simulink model "tp414070"  (Simulink 3.0)
settings: Solver=ode1  SolverMode=SingleTasking  StartTime=0.0  StopTime=t_sim  FixedStep=Ts  RelTol=1e-3
values from neighbouring files (symbols this model uses):
  d_action_on = 1    [init_PID1_windupless_tune3.m]
  i_action_on = 1    [init_PID1_windupless_tune3.m]
  Ks = input('Put integrator gain value Ks = ')    [init_PI1_windupless.m]    (also in init_PID1_windupless_tune3.m)
  P = input('Put gain of P component = ')    [init_PI1_windupless.m]    (also in init_PID1_windupless_tune3.m; init_step_resp2.m = 2)
  T1 = input('Put time constant T1 value = ')    [init_PID1_windupless_tune3.m]
  Tfd = input('feasibility and filtration (T1/5) = ')    [init_PID1_windupless_tune3.m]
  Tfil = input('Put time constant Tfil of inner loop = ')    [init_PI1_windupless.m]    (also in init_PID1_windupless_tune3.m)
  Ts = 1    [init_PI1_windupless.m]    (also in init_PID1_windupless_tune3.m = 0.5; init_step_resp2.m = 0.2; prev45_0.mat = 0.2; prev45_1.mat = 0.2)
  Umax = 5    [init_PI1_windupless.m]    (also in init_PID1_windupless_tune3.m; init_step_resp2.m; prev45_0.mat; prev45_1.mat)
  Umin = 0    [init_PI1_windupless.m]    (also in init_PID1_windupless_tune3.m; init_step_resp2.m; prev45_0.mat; prev45_1.mat)
libraries: udaq28LT_lib x1
settings Model: LastModifiedBy=mato  ExtModeMexFile=rtwinext  ExtModeTrigDuration=100000  SaveFormat=Matrix  RTWSystemTargetFile=rtwin.tlc  RTWTemplateMakefile=rtwintmf  RTWOptions="-aCCOptimize=1 -aEnforceIntegerDowncast=1 -aExtMode=1 -aFoldNonRolledExpr=1 -aForceParamTrailComments=0 -aGenerateComments=1 -aGenerateReport=0 -aIncDataTypeInIds=0 -aIncHierarchyInIds=0 -aInlineInvariantSignals=0 -aInlinedPrmAccess=\"Literals\" -aLocalBlockOutputs=1 -aMaxRTWIdLen=31 -aPrefixModelToSubsysFcnNames=1 -aRTWVerbose=1 -aRebuildAll=1 -aRollThreshold=5 -aShowEliminatedStatements=1"

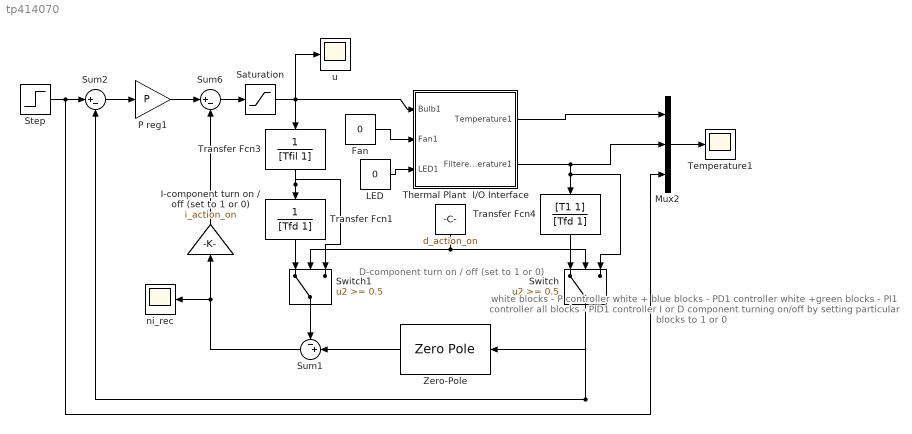
== system tp414070 ==
  note: D-component
      |  turn on / off
      | (set to 1 or 0)
  note: white blocks - P controller
      |
      | white + blue blocks - PD1 controller
      |
      | white +green blocks - PI1 controller
      |
      | all blocks - PID1 controller
      |
      |
      | I or D component turning on/off
      | by setting particular blocks to 1 or 0
  " " : Constant  Orientation=down  Value=d_action_on
  Fan : Constant  Value=0
  I-component turn on / off (set to 1 or 0) : Gain  Orientation=up  Gain=i_action_on  SaturateOnIntegerOverflow=on
  LED : Constant  Value=0
  Mux2 : Mux  Inputs=3
  P reg1 : Gain  Gain=P  SaturateOnIntegerOverflow=on
  Saturation : Saturate  UpperLimit=Umax  LowerLimit=Umin
  Step : Step  Time=0  Before=0  After=35  SampleTime=0
  Sum1 : Sum  Orientation=left  Inputs=-+|  SaturateOnIntegerOverflow=on
  Sum2 : Sum  Inputs=|+-  SaturateOnIntegerOverflow=on
  Sum6 : Sum  Inputs=|+-  SaturateOnIntegerOverflow=on
  Switch : Switch  Orientation=down  Threshold=0.5
  Switch1 : Switch  Orientation=down  Threshold=0.5
  Temperature1 : Scope
      settings: TickLabels=on  TimeRange=30  YMin=15  YMax=50  SaveName=yt  DataFormat=Matrix
  Thermal Plant  I/O Interface : Subsystem
      mask Display: disp('Thermo-optical\nPlant\nI/O Interface')
  Transfer Fcn1 : TransferFcn  Orientation=down  Numerator=[1]  Denominator=[Tfd 1]
  Transfer Fcn3 : TransferFcn  Orientation=down  Numerator=[1]  Denominator=[Tfil 1]
  Transfer Fcn4 : TransferFcn  Orientation=down  Numerator=[T1 1]  Denominator=[Tfd 1]
  Zero-Pole : ZeroPole  Orientation=left  Zeros=[0]  Poles=[-1/Tfil]  Gain=[1/(Ks*Tfil)]
  ni_rec : Scope
      settings: TimeRange=auto  YMin=1.5  YMax=2.7  SaveName=ni_rec  DataFormat=Matrix  Decimation=10  SampleInput=on  SampleTime=Ts
  u : Scope
      settings: TimeRange=180  YMin=0  YMax=5  SaveName=u  DataFormat=Matrix  Decimation=10  SampleInput=on  SampleTime=Ts
  wires:
  Sum2/1 -> P reg1/1
  Sum6/1 -> Saturation/1
  P reg1/1 -> Sum6/1
  Sum1/1 -> ni_rec/1, I-component turn on / off (set to 1 or 0)/1
  Step/1 -> Sum2/1, Mux2/3
  Saturation/1 -> Transfer Fcn3/1, u/1, Thermal Plant  I/O Interface/1(Bulb1)
  I-component turn on / off (set to 1 or 0)/1 -> Sum6/2
  Switch/1 -> Sum2/2, Zero-Pole/1
  Transfer Fcn4/1 -> Switch/1
  " "/1 -> Switch/2, Switch1/2
  Transfer Fcn3/1 -> Switch1/3, Transfer Fcn1/1
  Transfer Fcn1/1 -> Switch1/1
  Switch1/1 -> Sum1/1
  Zero-Pole/1 -> Sum1/2
  Mux2/1 -> Temperature1/1
  Fan/1 -> Thermal Plant  I/O Interface/2(Fan1)
  LED/1 -> Thermal Plant  I/O Interface/3(LED1)
  Thermal Plant  I/O Interface/1(Temperature1) -> Mux2/1
  Thermal Plant  I/O Interface/2(Filtered  temperature1) -> Mux2/2, Transfer Fcn4/1, Switch/3

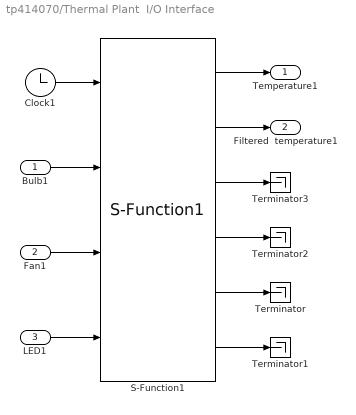
== system tp414070/Thermal Plant  I/O Interface ==
  Bulb1 : Inport  Port=1  PortWidth=-1  SampleTime=-1  DataType=auto
      settings: SignalType=auto
  Fan1 : Inport  Port=2  PortWidth=-1  SampleTime=-1  DataType=auto
      settings: SignalType=auto
  LED1 : Inport  Port=3  PortWidth=-1  SampleTime=-1  DataType=auto
      settings: SignalType=auto
  Clock1 : Clock
      settings: DisplayTime=off  Decimation=10
  S-Function1 : udaq28LT_lib/S-Function1  Priority=1  com_port=COM3  Ts=Ts  events_ot=2  rd_timeout=Ts/2*1000  matlab_prior=ABOVE_NORMAL_PRIORITY  warning=on  printout=off
  Terminator{,1..3} (4 alike) : Terminator
  Temperature1 : Outport  Port=1
  Filtered  temperature1 : Outport  Port=2
  wires:
  S-Function1/1 -> Temperature1/1
  S-Function1/2 -> Filtered  temperature1/1
  Clock1/1 -> S-Function1/1
  Bulb1/1 -> S-Function1/2
  Fan1/1 -> S-Function1/3
  S-Function1/3 -> Terminator3/1
  S-Function1/4 -> Terminator2/1
  S-Function1/5 -> Terminator/1
  S-Function1/6 -> Terminator1/1
  LED1/1 -> S-Function1/4
